simulink model "Model2_PLL"  (R2021b)
settings: Solver=ode45  StartTime=0.0  StopTime=100  MaxStep=1e-4  RelTol=1e-4  EnableMultiTasking=on
libraries: spspowerguiLib x1
settings Model: Creator=edu  LastModifiedBy=eprieto
settings SolverCC: AlgebraicLoopSolver=TrustRegion
settings DataIOCC: LimitDataPoints=on  SaveFormat=Array  SignalLoggingSaveFormat=ModelDataLogs  ReturnWorkspaceOutputs=off
settings OptimizationCC: ExpressionDepthLimit=2147483647  LifeSpan=inf
settings DebuggingCC: UnderspecifiedInitializationDetection=Classic  MergeDetectMultiDrivingBlocksExec=none  SolverPrmCheckMsg=warning  FcnCallInpInsideContextMsg=warning  StateNameClashWarn=warning  SFUnexpectedBacktrackingDiag=warning  SFNoUnconditionalDefaultTransitionDiag=warning  SFExecutionAtInitializationDiag=none  SFMachineParentedDataDiag=warning  ArithmeticOperatorsInVariantConditions=warning
settings HardwareCC: ProdBitPerPointer=32  ProdBitPerSizeT=32  ProdBitPerPtrDiffT=32  ProdLargestAtomicFloat=None  ProdIntDivRoundTo=Undefined  ProdEndianess=Unspecified  ProdWordSize=32  ProdHWDeviceType=32-bit Generic
settings ModelReferenceCC: PropagateSignalLabelsOutOfModel=off
settings SFSimCC: SimUseLocalCustomCode=off  CustomCodeUndefinedFunction=UseInterfaceOnly
settings RTWCC: RTWUseLocalCustomCode=off
settings CodeAppCC: StateflowObjectComments=on
settings GRTTargetCC: TargetLangStandard=C89/C90 (ANSI)  CombineOutputUpdateFcns=off  GRTInterface=on
settings ConfigComp: CovMetricSettings=dw  CovSaveCumulativeToWorkspaceVar=on  CovSaveSingleToWorkspaceVar=on  CovExternalEMLEnable=off
settings SimscapeCC: SimscapeNormalizeSystem=off
settings ConfigurationSet: Description=SimMechanics 2G

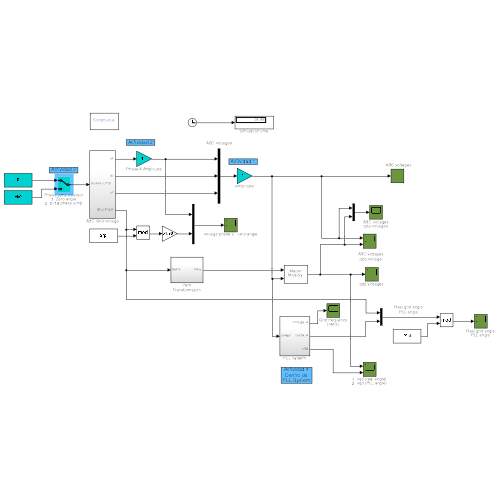
[thumbnail: Simulink's stored preview of the top-level diagram]
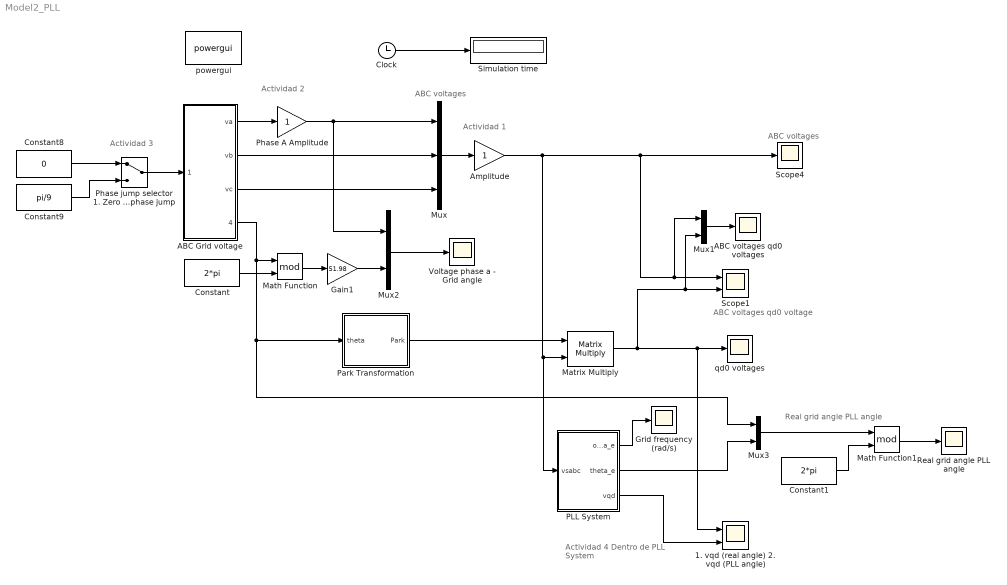
== system Model2_PLL ==
  note: Real grid angle
      | PLL angle
  note: ABC voltages
      | qd0 voltage
  note: ABC voltages
  note: ABC voltages
  note: Actividad 1
  note: Actividad 2
  note: Actividad 3
  note: Actividad 4
      | Dentro de
      | PLL System
  1. vqd (real angle) 2. vqd (PLL angle) : Scope  NumInputPorts=2
  ABC Grid voltage : Subsystem
  ABC voltages qd0 voltages : Scope
  Amplitude : Gain
  Clock : Clock
  Constant : Constant  Value=2*pi
  Constant1 : Constant  Value=2*pi
  Constant8 : Constant  Value=0
  Constant9 : Constant  Value=pi/9
  Gain1 : Gain  Gain=51.98
  Grid frequency (rad/s) : Scope
  Math Function : Math  Operator=mod  SignedPower=on  SaturateOnIntegerOverflow=on
  Math Function1 : Math  Operator=mod  SignedPower=on  SaturateOnIntegerOverflow=on
  Matrix Multiply : Product  Multiplication=Matrix(*)
  Mux : Mux  Inputs=3
  Mux1 : Mux  Inputs=2
  Mux2 : Mux  Inputs=2
  Mux3 : Mux  Inputs=2
  PLL System : Subsystem
  Park Transformation : Subsystem
  Phase A Amplitude : Gain
  Phase jump selector 1. Zero angle 2. pi/18 phase jump : ManualSwitch
  Real grid angle PLL angle : Scope
  Scope1 : Scope  NumInputPorts=2
  Scope4 : Scope
  Simulation time : Display
  Voltage phase a - Grid angle : Scope
  powergui : spspowerguiLib/powergui  Priority=1  SimulationMode=Continuous  SampleTime=50e-6  frequency=60  Iterations=50  frequencyindice=0  Pbase=100e6  ErrMax=1e-4  UnitsV=kV  UnitsW=MW  buscounter=0  FunctionMessages=off  echomessages=off  EnableUseOfTLC=off  CurrentSourceSwitches=on  DisableSnubberDevices=off  DisableRonSwitches=off  DisableVfSwitches=off  DisplayEquations=off  AutomaticDiscreteSolvers=off  SolverType=Tustin  Interpol=off  ExternalGateDelay=off  methode=off  Ts=0  x0status=blocks  SPID=off  SwTol=0  HookPort=off  NonlinearTolerance=1e-4  nMaxIteration=100  ContinueOnMaxIteration=off  RestoreLinks=warning  ResistiveCurrentMeasurement=off  Frange=[0:2:500]  Ylog=off  Xlog=on  ShowGrid=off  save=off  variable=ZData  structure=0  ZoomFFT=off  StartTime=0.0  cycles=1  DisplayStyle=1  fundamental=60  FreqAxis=off  MaxFrequency=1000  frequencyindicesteady=1  RmsSteady=1  display=off
  qd0 voltages : Scope
  wires:
  Mux/1 -> Amplitude/1
  Clock/1 -> Simulation time/1
  Park Transformation/1(Park) -> Matrix Multiply/1
  Matrix Multiply/1 -> 1. vqd (real angle) 2. vqd (PLL angle)/1, qd0 voltages/1, Scope1/2, Mux1/2
  Mux1/1 -> ABC voltages qd0 voltages/1
  ABC Grid voltage/1(va) -> Phase A Amplitude/1
  ABC Grid voltage/2(vb) -> Mux/2
  ABC Grid voltage/3(vc) -> Mux/3
  Mux2/1 -> Voltage phase a - Grid angle/1
  Math Function/1 -> Gain1/1
  Constant/1 -> Math Function/2
  Gain1/1 -> Mux2/2
  ABC Grid voltage/4(grid angle) -> Park Transformation/1(theta), Mux3/1, Math Function/1
  PLL System/3(vqd) -> 1. vqd (real angle) 2. vqd (PLL angle)/2
  PLL System/2(theta_e) -> Mux3/2
  Mux3/1 -> Math Function1/1
  Amplitude/1 -> Scope4/1, Scope1/1, Mux1/1, PLL System/1(vsabc), Matrix Multiply/2
  Constant1/1 -> Math Function1/2
  Math Function1/1 -> Real grid angle PLL angle/1
  Constant8/1 -> Phase jump selector 1. Zero angle 2. pi/18 phase jump/1
  Constant9/1 -> Phase jump selector 1. Zero angle 2. pi/18 phase jump/2
  Phase jump selector 1. Zero angle 2. pi/18 phase jump/1 -> ABC Grid voltage/1(Phase jump)
  PLL System/1(omega_e) -> Grid frequency (rad/s)/1
  Phase A Amplitude/1 -> Mux2/1, Mux/1

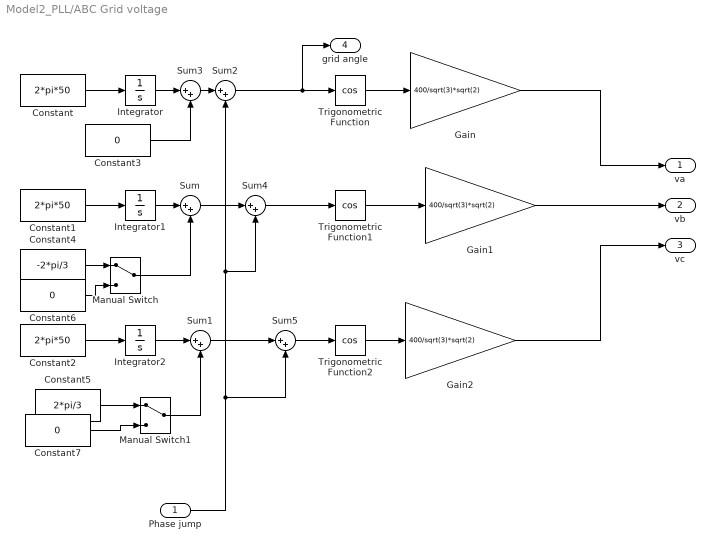
== system Model2_PLL/ABC Grid voltage ==
  Phase jump : Inport
  Constant : Constant  Value=2*pi*50
  Constant1 : Constant  Value=2*pi*50
  Constant2 : Constant  Value=2*pi*50
  Constant3 : Constant  Value=0
  Constant4 : Constant  Value=-2*pi/3
  Constant5 : Constant  Value=2*pi/3
  Constant6 : Constant  Value=0
  Constant7 : Constant  Value=0
  Gain : Gain  Gain=400/sqrt(3)*sqrt(2)
  Gain1 : Gain  Gain=400/sqrt(3)*sqrt(2)
  Gain2 : Gain  Gain=400/sqrt(3)*sqrt(2)
  Integrator : Integrator
  Integrator1 : Integrator
  Integrator2 : Integrator
  Manual Switch : ManualSwitch
  Manual Switch1 : ManualSwitch
  Sum{,1..5} (6 alike) : Sum  Inputs=|++
  Trigonometric Function : Trigonometry  Operator=cos
  Trigonometric Function1 : Trigonometry  Operator=cos
  Trigonometric Function2 : Trigonometry  Operator=cos
  va : Outport
  vb : Outport  Port=2
  vc : Outport  Port=3
  grid angle : Outport  Port=4
  wires:
  Constant2/1 -> Integrator2/1
  Integrator2/1 -> Sum1/1
  Gain2/1 -> vc/1
  Sum5/1 -> Trigonometric Function2/1
  Sum2/1 -> grid angle/1, Trigonometric Function/1
  Integrator/1 -> Sum3/1
  Manual Switch1/1 -> Sum1/2
  Manual Switch/1 -> Sum/2
  Integrator1/1 -> Sum/1
  Trigonometric Function/1 -> Gain/1
  Gain/1 -> va/1
  Constant1/1 -> Integrator1/1
  Trigonometric Function2/1 -> Gain2/1
  Constant/1 -> Integrator/1
  Constant3/1 -> Sum3/2
  Trigonometric Function1/1 -> Gain1/1
  Gain1/1 -> vb/1
  Sum4/1 -> Trigonometric Function1/1
  Constant4/1 -> Manual Switch/1
  Constant6/1 -> Manual Switch/2
  Constant5/1 -> Manual Switch1/1
  Constant7/1 -> Manual Switch1/2
  Sum3/1 -> Sum2/1
  Sum/1 -> Sum4/1
  Sum1/1 -> Sum5/1
  Phase jump/1 -> Sum5/2, Sum4/2, Sum2/2

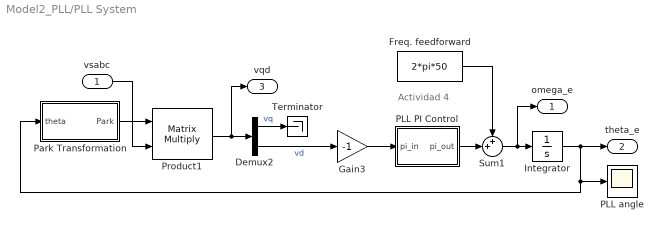
== system Model2_PLL/PLL System ==
  note: Actividad 4
  vsabc : Inport
  Demux2 : Demux  Outputs=2
  Freq. feedforward : Constant  Value=2*pi*50
  Gain3 : Gain  Gain=-1
  Integrator : Integrator
  PLL PI Control : Subsystem
  PLL angle : Scope
  Park Transformation : Subsystem
  Product1 : Product  Multiplication=Matrix(*)  RndMeth=Zero
  Sum1 : Sum  Inputs=++|
  Terminator : Terminator
  omega_e : Outport
  theta_e : Outport  Port=2
  vqd : Outport  Port=3
  wires:
  Integrator/1 -> theta_e/1, PLL angle/1, Park Transformation/1(theta)
  Park Transformation/1(Park) -> Product1/1
  Demux2/2 -> Gain3/1  "vd"
  Sum1/1 -> Integrator/1, omega_e/1
  Freq. feedforward/1 -> Sum1/1
  vsabc/1 -> Product1/2
  Product1/1 -> vqd/1, Demux2/1
  Gain3/1 -> PLL PI Control/1(pi_in)
  PLL PI Control/1(pi_out) -> Sum1/2
  Demux2/1 -> Terminator/1  "vq"

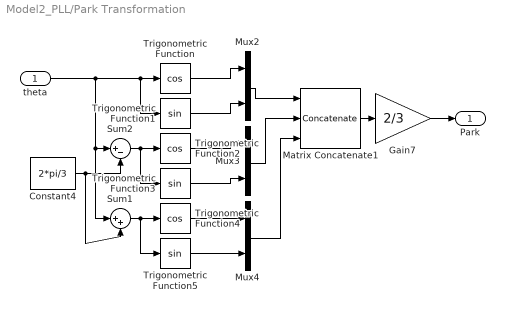
== system Model2_PLL/Park Transformation ==
  theta : Inport  PortDimensions=1
  Constant4 : Constant  Value=2*pi/3  SampleTime=-1
  Gain7 : Gain  Gain=2/3
  Matrix Concatenate1 : Concatenate  NumInputs=3  Mode=Multidimensional array  ConcatenateDimension=2
  Mux2 : Mux  Inputs=2
  Mux3 : Mux  Inputs=2
  Mux4 : Mux  Inputs=2
  Sum1 : Sum  Inputs=|++
  Sum2 : Sum  Inputs=|+-
  Trigonometric Function : Trigonometry  Operator=cos
  Trigonometric Function1 : Trigonometry
  Trigonometric Function2 : Trigonometry  Operator=cos
  Trigonometric Function3 : Trigonometry
  Trigonometric Function4 : Trigonometry  Operator=cos
  Trigonometric Function5 : Trigonometry
  Park : Outport
  wires:
  theta/1 -> Sum1/1, Sum2/1, Trigonometric Function/1, Trigonometric Function1/1
  Sum2/1 -> Trigonometric Function2/1, Trigonometric Function3/1
  Sum1/1 -> Trigonometric Function4/1, Trigonometric Function5/1
  Constant4/1 -> Sum2/2, Sum1/2
  Trigonometric Function/1 -> Mux2/1
  Trigonometric Function1/1 -> Mux2/2
  Trigonometric Function2/1 -> Mux3/1
  Trigonometric Function3/1 -> Mux3/2
  Trigonometric Function4/1 -> Mux4/1
  Trigonometric Function5/1 -> Mux4/2
  Mux2/1 -> Matrix Concatenate1/1
  Mux3/1 -> Matrix Concatenate1/2
  Mux4/1 -> Matrix Concatenate1/3
  Matrix Concatenate1/1 -> Gain7/1
  Gain7/1 -> Park/1

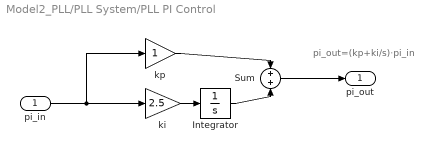
== system Model2_PLL/PLL System/PLL PI Control ==
  note: pi_out=(kp+ki/s)·pi_in
  pi_in : Inport
  Integrator : Integrator
  Sum : Sum
  ki : Gain  Gain=2.5
  kp : Gain
  pi_out : Outport
  wires:
  Sum/1 -> pi_out/1
  Integrator/1 -> Sum/2
  ki/1 -> Integrator/1
  kp/1 -> Sum/1
  pi_in/1 -> ki/1, kp/1

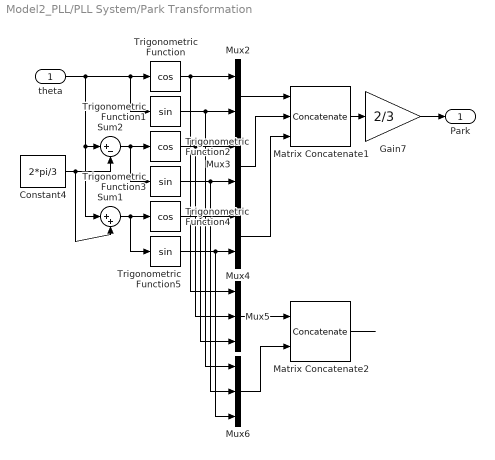
== system Model2_PLL/PLL System/Park Transformation ==
  theta : Inport  PortDimensions=1
  Constant4 : Constant  Value=2*pi/3  SampleTime=-1
  Gain7 : Gain  Gain=2/3
  Matrix Concatenate1 : Concatenate  NumInputs=3  Mode=Multidimensional array  ConcatenateDimension=2
  Matrix Concatenate2 : Concatenate  Mode=Multidimensional array  ConcatenateDimension=2
  Mux2 : Mux  Inputs=2
  Mux3 : Mux  Inputs=2
  Mux4 : Mux  Inputs=2
  Mux5 : Mux  Inputs=3
  Mux6 : Mux  Inputs=3
  Sum1 : Sum  Inputs=|++
  Sum2 : Sum  Inputs=|+-
  Trigonometric Function : Trigonometry  Operator=cos
  Trigonometric Function1 : Trigonometry
  Trigonometric Function2 : Trigonometry  Operator=cos
  Trigonometric Function3 : Trigonometry
  Trigonometric Function4 : Trigonometry  Operator=cos
  Trigonometric Function5 : Trigonometry
  Park : Outport
  wires:
  theta/1 -> Sum1/1, Sum2/1, Trigonometric Function/1, Trigonometric Function1/1
  Sum2/1 -> Trigonometric Function2/1, Trigonometric Function3/1
  Sum1/1 -> Trigonometric Function4/1, Trigonometric Function5/1
  Constant4/1 -> Sum2/2, Sum1/2
  Trigonometric Function/1 -> Mux2/1, Mux5/1
  Trigonometric Function1/1 -> Mux2/2, Mux6/1
  Trigonometric Function2/1 -> Mux3/1, Mux5/2
  Trigonometric Function3/1 -> Mux3/2, Mux6/2
  Trigonometric Function4/1 -> Mux4/1, Mux5/3
  Trigonometric Function5/1 -> Mux4/2, Mux6/3
  Mux2/1 -> Matrix Concatenate1/1
  Mux3/1 -> Matrix Concatenate1/2
  Mux4/1 -> Matrix Concatenate1/3
  Matrix Concatenate1/1 -> Gain7/1
  Mux5/1 -> Matrix Concatenate2/1
  Mux6/1 -> Matrix Concatenate2/2
  Gain7/1 -> Park/1
  Matrix Concatenate2/1 -> ?
